simulink model "AxialPump_23a"  (R2023a)
settings: Solver=FixedStepAuto  StartTime=0.0  StopTime=t_cycle  FixedStep=1e-8  RelTol=1e-3  EnableMultiTasking=on
InitFcn:
  | %% Outlet
  | % Parameters
  | d_cyl = 8e-3;                                   % Diameter of each piston
  | r_p = 20e-3;                                    % Piston pitch radius
  | A_cyl = 0.25 * pi * d_cyl^2;                    % Area of each piston
  | omega_rpm = 3600;                               % Rotational speed of pump
  | omega = (2*pi/60) * omega_rpm;                  % Angular speed of pump
  | beta = 1.6e9;                                   % Bulk Modulus
  | P1 = 21e6;                                      % Outlet pressure
  | S = 15e-3;                                      % Stroke length
  | Cd = 0.6;                                       % Coefficient of discharge
  | rho = 870;                                      % Density
  | P_T = 101325;                                   % Tank pressure
  | P_P = 21e6;                                     % System pressure
  | c = 80e-6;                                      % Piston-barrel clearance
  | meu = 0.1;                                      % Steel-steel (lubricated) coefficient of friction
  | r2_r1 = 1.6;                                    % Slipper radii ratio
  | r1 = d_cyl/2;
  | do = 0.1e-3;                                    % Slipper orifice opening
  | 
  | % Time parameters
  | theta_cycle = 2 * pi;
  | t_cycle = theta_cycle / omega;
  | theta_t = 2 * asin(d_cyl/(4*r_p));
  | t_t = theta_t/omega;
  | theta_d = theta_cycle/2 - 2 * theta_t;
  | t_d = theta_d/omega;
  | 
  | t_A_p = [0, 0.5*t_t, t_t, t_t+t_d, 1.5*t_t+t_d, t_cycle];
  | A_p = [0, 0, A_cyl, A_cyl, 0, 0];
  | 
  | t_A_t = [0, 2.5*t_t+t_d, 3*t_t+t_d, 3*t_t+2*t_d, 3.5*t_t+2*t_d, t_cycle];
  | A_t = [0, 0, A_cyl, A_cyl, 0, 0];
  | 
  | % Calculated parameters
  | Vdisp = 0.25 * pi * d_cyl^2 * S;
  | Vo = Vdisp;
libraries: SignalEditorBlockLib x18
(part 2 of 2)

== system AxialPump_23a/Piston 2/Full Throttling Loss (Tank Side) ==
  Pc : Inport
  P_T : Inport  Port=2
  Q_T : Inport  Port=3
  Display : Display
  Integrator : Integrator
  MATLAB Function : MATLAB Function  TreatAsAtomicUnit=on
  Scope : Scope
  " E_ftlts" : Outport
  wires:
  MATLAB Function/1(P_ftlts) -> Scope/1, Integrator/1
  Integrator/1 -> Display/1, " E_ftlts"/1  "E_ftlts"
  Pc/1 -> MATLAB Function/2(Pc)
  P_T/1 -> MATLAB Function/1(P_T)
  Q_T/1 -> MATLAB Function/3(Q_T)

== system AxialPump_23a/Piston 2/Hydrostatic Bearing Loss ==
  Pc : Inport
  Constant : Constant  Value=Cd
  Constant1 : Constant  Value=r2_r1
  Constant2 : Constant  Value=r1
  Constant3 : Constant  Value=do
  Constant4 : Constant  Value=d_cyl
  Constant5 : Constant  Value=rho
  Display : Display
  Integrator : Integrator
  MATLAB Function : MATLAB Function  TreatAsAtomicUnit=on
  Product : Product
  Ehbl : Outport
  wires:
  Constant1/1 -> MATLAB Function/2(r2_r1)
  Constant/1 -> MATLAB Function/6(Cd)
  Constant4/1 -> MATLAB Function/5(d_cyl)
  Constant3/1 -> MATLAB Function/4(do)
  Constant2/1 -> MATLAB Function/3(r1)
  Pc/1 -> Product/2, MATLAB Function/7(Pc)
  MATLAB Function/1(Qhbl) -> Product/1
  Product/1 -> Integrator/1  "Phbl"
  Integrator/1 -> Display/1, Ehbl/1
  Constant5/1 -> MATLAB Function/1(rho)

== system AxialPump_23a/Piston 2/Qleak ==
  Pc : Inport
  Constant : Constant  Value=P_T
  Constant1 : Constant  Value=d_cyl
  Constant2 : Constant  Value=c
  Constant3 : Constant  Value=meu
  Constant4 : Constant  Value=S
  Display : Display
  Integrator2 : Integrator
  MATLAB Function : MATLAB Function  TreatAsAtomicUnit=on
  Product1 : Product
  Eleak : Outport
  wires:
  Constant/1 -> MATLAB Function/2(P_T)
  Constant1/1 -> MATLAB Function/3(d_cyl)
  Constant2/1 -> MATLAB Function/4(c)
  Constant3/1 -> MATLAB Function/5(meu)
  Constant4/1 -> MATLAB Function/6(S)
  Pc/1 -> MATLAB Function/1(Pc), Product1/2
  MATLAB Function/1(Qleak) -> Product1/1
  Integrator2/1 -> Display/1, Eleak/1
  Product1/1 -> Integrator2/1  "Pleakage"

== system AxialPump_23a/Piston 3/Frictional Energy Loss ==
  Vc_dot : Inport
  Vc : Inport  Port=2
  Constant : Constant  Value=Vo
  Constant1 : Constant  Value=A_cyl
  Constant2 : Constant  Value=S
  Constant3 : Constant  Value=c
  Constant4 : Constant  Value=meu
  Constant5 : Constant  Value=d_cyl
  Frictional Energy Loss : Display
  Gain : Gain  Gain=1/A_cyl
  Integrator : Integrator
  MATLAB Function : MATLAB Function  TreatAsAtomicUnit=on
  Scope : Scope
  Efric : Outport
  wires:
  Integrator/1 -> Frictional Energy Loss/1, Efric/1
  Vc_dot/1 -> Gain/1
  Gain/1 -> MATLAB Function/1(xdot)  "xdot"
  MATLAB Function/1(Pfric) -> Integrator/1  "Pfric"
  MATLAB Function/2(x) -> Scope/1  "x"
  Vc/1 -> MATLAB Function/2(Vc)
  Constant/1 -> MATLAB Function/3(Vo)
  Constant1/1 -> MATLAB Function/4(A_cyl)
  Constant2/1 -> MATLAB Function/5(S)
  Constant3/1 -> MATLAB Function/6(c)
  Constant4/1 -> MATLAB Function/7(meu)
  Constant5/1 -> MATLAB Function/8(d_cyl)

== system AxialPump_23a/Piston 3/Full Throttling Loss (Pressure Side) ==
  Pc : Inport
  P_P : Inport  Port=2
  Q_P : Inport  Port=3
  Display : Display
  Integrator : Integrator
  MATLAB Function : MATLAB Function  TreatAsAtomicUnit=on
  Scope : Scope
  " E_ftlps" : Outport
  wires:
  MATLAB Function/1(P_ftlps) -> Scope/1, Integrator/1
  Integrator/1 -> Display/1, " E_ftlps"/1  "E_ftlps"
  Pc/1 -> MATLAB Function/1(Pc)
  P_P/1 -> MATLAB Function/2(P_P)
  Q_P/1 -> MATLAB Function/3(Q_P)

== system AxialPump_23a/Piston 3/Full Throttling Loss (Tank Side) ==
  Pc : Inport
  P_T : Inport  Port=2
  Q_T : Inport  Port=3
  Display : Display
  Integrator : Integrator
  MATLAB Function : MATLAB Function  TreatAsAtomicUnit=on
  Scope : Scope
  " E_ftlts" : Outport
  wires:
  MATLAB Function/1(P_ftlts) -> Scope/1, Integrator/1
  Integrator/1 -> Display/1, " E_ftlts"/1  "E_ftlts"
  Pc/1 -> MATLAB Function/2(Pc)
  P_T/1 -> MATLAB Function/1(P_T)
  Q_T/1 -> MATLAB Function/3(Q_T)

== system AxialPump_23a/Piston 3/Hydrostatic Bearing Loss ==
  Pc : Inport
  Constant : Constant  Value=Cd
  Constant1 : Constant  Value=r2_r1
  Constant2 : Constant  Value=r1
  Constant3 : Constant  Value=do
  Constant4 : Constant  Value=d_cyl
  Constant5 : Constant  Value=rho
  Display : Display
  Integrator : Integrator
  MATLAB Function : MATLAB Function  TreatAsAtomicUnit=on
  Product : Product
  Ehbl : Outport
  wires:
  Constant1/1 -> MATLAB Function/2(r2_r1)
  Constant/1 -> MATLAB Function/6(Cd)
  Constant4/1 -> MATLAB Function/5(d_cyl)
  Constant3/1 -> MATLAB Function/4(do)
  Constant2/1 -> MATLAB Function/3(r1)
  Pc/1 -> Product/2, MATLAB Function/7(Pc)
  MATLAB Function/1(Qhbl) -> Product/1
  Product/1 -> Integrator/1  "Phbl"
  Integrator/1 -> Display/1, Ehbl/1
  Constant5/1 -> MATLAB Function/1(rho)

== system AxialPump_23a/Piston 3/Qleak ==
  Pc : Inport
  Constant : Constant  Value=P_T
  Constant1 : Constant  Value=d_cyl
  Constant2 : Constant  Value=c
  Constant3 : Constant  Value=meu
  Constant4 : Constant  Value=S
  Display : Display
  Integrator2 : Integrator
  MATLAB Function : MATLAB Function  TreatAsAtomicUnit=on
  Product1 : Product
  Eleak : Outport
  wires:
  Constant/1 -> MATLAB Function/2(P_T)
  Constant1/1 -> MATLAB Function/3(d_cyl)
  Constant2/1 -> MATLAB Function/4(c)
  Constant3/1 -> MATLAB Function/5(meu)
  Constant4/1 -> MATLAB Function/6(S)
  Pc/1 -> MATLAB Function/1(Pc), Product1/2
  MATLAB Function/1(Qleak) -> Product1/1
  Integrator2/1 -> Display/1, Eleak/1
  Product1/1 -> Integrator2/1  "Pleakage"

== system AxialPump_23a/Piston 4/Frictional Energy Loss ==
  Vc_dot : Inport
  Vc : Inport  Port=2
  Constant : Constant  Value=Vo
  Constant1 : Constant  Value=A_cyl
  Constant2 : Constant  Value=S
  Constant3 : Constant  Value=c
  Constant4 : Constant  Value=meu
  Constant5 : Constant  Value=d_cyl
  Frictional Energy Loss : Display
  Gain : Gain  Gain=1/A_cyl
  Integrator : Integrator
  MATLAB Function : MATLAB Function  TreatAsAtomicUnit=on
  Scope : Scope
  Efric : Outport
  wires:
  Integrator/1 -> Frictional Energy Loss/1, Efric/1
  Vc_dot/1 -> Gain/1
  Gain/1 -> MATLAB Function/1(xdot)  "xdot"
  MATLAB Function/1(Pfric) -> Integrator/1  "Pfric"
  MATLAB Function/2(x) -> Scope/1  "x"
  Vc/1 -> MATLAB Function/2(Vc)
  Constant/1 -> MATLAB Function/3(Vo)
  Constant1/1 -> MATLAB Function/4(A_cyl)
  Constant2/1 -> MATLAB Function/5(S)
  Constant3/1 -> MATLAB Function/6(c)
  Constant4/1 -> MATLAB Function/7(meu)
  Constant5/1 -> MATLAB Function/8(d_cyl)

== system AxialPump_23a/Piston 4/Full Throttling Loss (Pressure Side) ==
  Pc : Inport
  P_P : Inport  Port=2
  Q_P : Inport  Port=3
  Display : Display
  Integrator : Integrator
  MATLAB Function : MATLAB Function  TreatAsAtomicUnit=on
  Scope : Scope
  " E_ftlps" : Outport
  wires:
  MATLAB Function/1(P_ftlps) -> Scope/1, Integrator/1
  Integrator/1 -> Display/1, " E_ftlps"/1  "E_ftlps"
  Pc/1 -> MATLAB Function/1(Pc)
  P_P/1 -> MATLAB Function/2(P_P)
  Q_P/1 -> MATLAB Function/3(Q_P)

== system AxialPump_23a/Piston 4/Full Throttling Loss (Tank Side) ==
  Pc : Inport
  P_T : Inport  Port=2
  Q_T : Inport  Port=3
  Display : Display
  Integrator : Integrator
  MATLAB Function : MATLAB Function  TreatAsAtomicUnit=on
  Scope : Scope
  " E_ftlts" : Outport
  wires:
  MATLAB Function/1(P_ftlts) -> Scope/1, Integrator/1
  Integrator/1 -> Display/1, " E_ftlts"/1  "E_ftlts"
  Pc/1 -> MATLAB Function/2(Pc)
  P_T/1 -> MATLAB Function/1(P_T)
  Q_T/1 -> MATLAB Function/3(Q_T)

== system AxialPump_23a/Piston 4/Hydrostatic Bearing Loss ==
  Pc : Inport
  Constant : Constant  Value=Cd
  Constant1 : Constant  Value=r2_r1
  Constant2 : Constant  Value=r1
  Constant3 : Constant  Value=do
  Constant4 : Constant  Value=d_cyl
  Constant5 : Constant  Value=rho
  Display : Display
  Integrator : Integrator
  MATLAB Function : MATLAB Function  TreatAsAtomicUnit=on
  Product : Product
  Ehbl : Outport
  wires:
  Constant1/1 -> MATLAB Function/2(r2_r1)
  Constant/1 -> MATLAB Function/6(Cd)
  Constant4/1 -> MATLAB Function/5(d_cyl)
  Constant3/1 -> MATLAB Function/4(do)
  Constant2/1 -> MATLAB Function/3(r1)
  Pc/1 -> Product/2, MATLAB Function/7(Pc)
  MATLAB Function/1(Qhbl) -> Product/1
  Product/1 -> Integrator/1  "Phbl"
  Integrator/1 -> Display/1, Ehbl/1
  Constant5/1 -> MATLAB Function/1(rho)

== system AxialPump_23a/Piston 4/Qleak ==
  Pc : Inport
  Constant : Constant  Value=P_T
  Constant1 : Constant  Value=d_cyl
  Constant2 : Constant  Value=c
  Constant3 : Constant  Value=meu
  Constant4 : Constant  Value=S
  Display : Display
  Integrator2 : Integrator
  MATLAB Function : MATLAB Function  TreatAsAtomicUnit=on
  Product1 : Product
  Eleak : Outport
  wires:
  Constant/1 -> MATLAB Function/2(P_T)
  Constant1/1 -> MATLAB Function/3(d_cyl)
  Constant2/1 -> MATLAB Function/4(c)
  Constant3/1 -> MATLAB Function/5(meu)
  Constant4/1 -> MATLAB Function/6(S)
  Pc/1 -> MATLAB Function/1(Pc), Product1/2
  MATLAB Function/1(Qleak) -> Product1/1
  Integrator2/1 -> Display/1, Eleak/1
  Product1/1 -> Integrator2/1  "Pleakage"

== system AxialPump_23a/Piston 5/Frictional Energy Loss ==
  Vc_dot : Inport
  Vc : Inport  Port=2
  Constant : Constant  Value=Vo
  Constant1 : Constant  Value=A_cyl
  Constant2 : Constant  Value=S
  Constant3 : Constant  Value=c
  Constant4 : Constant  Value=meu
  Constant5 : Constant  Value=d_cyl
  Frictional Energy Loss : Display
  Gain : Gain  Gain=1/A_cyl
  Integrator : Integrator
  MATLAB Function : MATLAB Function  TreatAsAtomicUnit=on
  Scope : Scope
  Efric : Outport
  wires:
  Integrator/1 -> Frictional Energy Loss/1, Efric/1
  Vc_dot/1 -> Gain/1
  Gain/1 -> MATLAB Function/1(xdot)  "xdot"
  MATLAB Function/1(Pfric) -> Integrator/1  "Pfric"
  MATLAB Function/2(x) -> Scope/1  "x"
  Vc/1 -> MATLAB Function/2(Vc)
  Constant/1 -> MATLAB Function/3(Vo)
  Constant1/1 -> MATLAB Function/4(A_cyl)
  Constant2/1 -> MATLAB Function/5(S)
  Constant3/1 -> MATLAB Function/6(c)
  Constant4/1 -> MATLAB Function/7(meu)
  Constant5/1 -> MATLAB Function/8(d_cyl)

== system AxialPump_23a/Piston 5/Full Throttling Loss (Pressure Side) ==
  Pc : Inport
  P_P : Inport  Port=2
  Q_P : Inport  Port=3
  Display : Display
  Integrator : Integrator
  MATLAB Function : MATLAB Function  TreatAsAtomicUnit=on
  Scope : Scope
  " E_ftlps" : Outport
  wires:
  MATLAB Function/1(P_ftlps) -> Scope/1, Integrator/1
  Integrator/1 -> Display/1, " E_ftlps"/1  "E_ftlps"
  Pc/1 -> MATLAB Function/1(Pc)
  P_P/1 -> MATLAB Function/2(P_P)
  Q_P/1 -> MATLAB Function/3(Q_P)

== system AxialPump_23a/Piston 5/Full Throttling Loss (Tank Side) ==
  Pc : Inport
  P_T : Inport  Port=2
  Q_T : Inport  Port=3
  Display : Display
  Integrator : Integrator
  MATLAB Function : MATLAB Function  TreatAsAtomicUnit=on
  Scope : Scope
  " E_ftlts" : Outport
  wires:
  MATLAB Function/1(P_ftlts) -> Scope/1, Integrator/1
  Integrator/1 -> Display/1, " E_ftlts"/1  "E_ftlts"
  Pc/1 -> MATLAB Function/2(Pc)
  P_T/1 -> MATLAB Function/1(P_T)
  Q_T/1 -> MATLAB Function/3(Q_T)

== system AxialPump_23a/Piston 5/Hydrostatic Bearing Loss ==
  Pc : Inport
  Constant : Constant  Value=Cd
  Constant1 : Constant  Value=r2_r1
  Constant2 : Constant  Value=r1
  Constant3 : Constant  Value=do
  Constant4 : Constant  Value=d_cyl
  Constant5 : Constant  Value=rho
  Display : Display
  Integrator : Integrator
  MATLAB Function : MATLAB Function  TreatAsAtomicUnit=on
  Product : Product
  Ehbl : Outport
  wires:
  Constant1/1 -> MATLAB Function/2(r2_r1)
  Constant/1 -> MATLAB Function/6(Cd)
  Constant4/1 -> MATLAB Function/5(d_cyl)
  Constant3/1 -> MATLAB Function/4(do)
  Constant2/1 -> MATLAB Function/3(r1)
  Pc/1 -> Product/2, MATLAB Function/7(Pc)
  MATLAB Function/1(Qhbl) -> Product/1
  Product/1 -> Integrator/1  "Phbl"
  Integrator/1 -> Display/1, Ehbl/1
  Constant5/1 -> MATLAB Function/1(rho)

== system AxialPump_23a/Piston 5/Qleak ==
  Pc : Inport
  Constant : Constant  Value=P_T
  Constant1 : Constant  Value=d_cyl
  Constant2 : Constant  Value=c
  Constant3 : Constant  Value=meu
  Constant4 : Constant  Value=S
  Display : Display
  Integrator2 : Integrator
  MATLAB Function : MATLAB Function  TreatAsAtomicUnit=on
  Product1 : Product
  Eleak : Outport
  wires:
  Constant/1 -> MATLAB Function/2(P_T)
  Constant1/1 -> MATLAB Function/3(d_cyl)
  Constant2/1 -> MATLAB Function/4(c)
  Constant3/1 -> MATLAB Function/5(meu)
  Constant4/1 -> MATLAB Function/6(S)
  Pc/1 -> MATLAB Function/1(Pc), Product1/2
  MATLAB Function/1(Qleak) -> Product1/1
  Integrator2/1 -> Display/1, Eleak/1
  Product1/1 -> Integrator2/1  "Pleakage"

== system AxialPump_23a/Piston 6/Frictional Energy Loss ==
  Vc_dot : Inport
  Vc : Inport  Port=2
  Constant : Constant  Value=Vo
  Constant1 : Constant  Value=A_cyl
  Constant2 : Constant  Value=S
  Constant3 : Constant  Value=c
  Constant4 : Constant  Value=meu
  Constant5 : Constant  Value=d_cyl
  Frictional Energy Loss : Display
  Gain : Gain  Gain=1/A_cyl
  Integrator : Integrator
  MATLAB Function : MATLAB Function  TreatAsAtomicUnit=on
  Scope : Scope
  Efric : Outport
  wires:
  Integrator/1 -> Frictional Energy Loss/1, Efric/1
  Vc_dot/1 -> Gain/1
  Gain/1 -> MATLAB Function/1(xdot)  "xdot"
  MATLAB Function/1(Pfric) -> Integrator/1  "Pfric"
  MATLAB Function/2(x) -> Scope/1  "x"
  Vc/1 -> MATLAB Function/2(Vc)
  Constant/1 -> MATLAB Function/3(Vo)
  Constant1/1 -> MATLAB Function/4(A_cyl)
  Constant2/1 -> MATLAB Function/5(S)
  Constant3/1 -> MATLAB Function/6(c)
  Constant4/1 -> MATLAB Function/7(meu)
  Constant5/1 -> MATLAB Function/8(d_cyl)

== system AxialPump_23a/Piston 6/Full Throttling Loss (Pressure Side) ==
  Pc : Inport
  P_P : Inport  Port=2
  Q_P : Inport  Port=3
  Display : Display
  Integrator : Integrator
  MATLAB Function : MATLAB Function  TreatAsAtomicUnit=on
  Scope : Scope
  " E_ftlps" : Outport
  wires:
  MATLAB Function/1(P_ftlps) -> Scope/1, Integrator/1
  Integrator/1 -> Display/1, " E_ftlps"/1  "E_ftlps"
  Pc/1 -> MATLAB Function/1(Pc)
  P_P/1 -> MATLAB Function/2(P_P)
  Q_P/1 -> MATLAB Function/3(Q_P)

== system AxialPump_23a/Piston 6/Full Throttling Loss (Tank Side) ==
  Pc : Inport
  P_T : Inport  Port=2
  Q_T : Inport  Port=3
  Display : Display
  Integrator : Integrator
  MATLAB Function : MATLAB Function  TreatAsAtomicUnit=on
  Scope : Scope
  " E_ftlts" : Outport
  wires:
  MATLAB Function/1(P_ftlts) -> Scope/1, Integrator/1
  Integrator/1 -> Display/1, " E_ftlts"/1  "E_ftlts"
  Pc/1 -> MATLAB Function/2(Pc)
  P_T/1 -> MATLAB Function/1(P_T)
  Q_T/1 -> MATLAB Function/3(Q_T)

== system AxialPump_23a/Piston 6/Hydrostatic Bearing Loss ==
  Pc : Inport
  Constant : Constant  Value=Cd
  Constant1 : Constant  Value=r2_r1
  Constant2 : Constant  Value=r1
  Constant3 : Constant  Value=do
  Constant4 : Constant  Value=d_cyl
  Constant5 : Constant  Value=rho
  Display : Display
  Integrator : Integrator
  MATLAB Function : MATLAB Function  TreatAsAtomicUnit=on
  Product : Product
  Ehbl : Outport
  wires:
  Constant1/1 -> MATLAB Function/2(r2_r1)
  Constant/1 -> MATLAB Function/6(Cd)
  Constant4/1 -> MATLAB Function/5(d_cyl)
  Constant3/1 -> MATLAB Function/4(do)
  Constant2/1 -> MATLAB Function/3(r1)
  Pc/1 -> Product/2, MATLAB Function/7(Pc)
  MATLAB Function/1(Qhbl) -> Product/1
  Product/1 -> Integrator/1  "Phbl"
  Integrator/1 -> Display/1, Ehbl/1
  Constant5/1 -> MATLAB Function/1(rho)

== system AxialPump_23a/Piston 6/Qleak ==
  Pc : Inport
  Constant : Constant  Value=P_T
  Constant1 : Constant  Value=d_cyl
  Constant2 : Constant  Value=c
  Constant3 : Constant  Value=meu
  Constant4 : Constant  Value=S
  Display : Display
  Integrator2 : Integrator
  MATLAB Function : MATLAB Function  TreatAsAtomicUnit=on
  Product1 : Product
  Eleak : Outport
  wires:
  Constant/1 -> MATLAB Function/2(P_T)
  Constant1/1 -> MATLAB Function/3(d_cyl)
  Constant2/1 -> MATLAB Function/4(c)
  Constant3/1 -> MATLAB Function/5(meu)
  Constant4/1 -> MATLAB Function/6(S)
  Pc/1 -> MATLAB Function/1(Pc), Product1/2
  MATLAB Function/1(Qleak) -> Product1/1
  Integrator2/1 -> Display/1, Eleak/1
  Product1/1 -> Integrator2/1  "Pleakage"

== system AxialPump_23a/Piston 7/Frictional Energy Loss ==
  Vc_dot : Inport
  Vc : Inport  Port=2
  Constant : Constant  Value=Vo
  Constant1 : Constant  Value=A_cyl
  Constant2 : Constant  Value=S
  Constant3 : Constant  Value=c
  Constant4 : Constant  Value=meu
  Constant5 : Constant  Value=d_cyl
  Frictional Energy Loss : Display
  Gain : Gain  Gain=1/A_cyl
  Integrator : Integrator
  MATLAB Function : MATLAB Function  TreatAsAtomicUnit=on
  Scope : Scope
  Efric : Outport
  wires:
  Integrator/1 -> Frictional Energy Loss/1, Efric/1
  Vc_dot/1 -> Gain/1
  Gain/1 -> MATLAB Function/1(xdot)  "xdot"
  MATLAB Function/1(Pfric) -> Integrator/1  "Pfric"
  MATLAB Function/2(x) -> Scope/1  "x"
  Vc/1 -> MATLAB Function/2(Vc)
  Constant/1 -> MATLAB Function/3(Vo)
  Constant1/1 -> MATLAB Function/4(A_cyl)
  Constant2/1 -> MATLAB Function/5(S)
  Constant3/1 -> MATLAB Function/6(c)
  Constant4/1 -> MATLAB Function/7(meu)
  Constant5/1 -> MATLAB Function/8(d_cyl)

== system AxialPump_23a/Piston 7/Full Throttling Loss (Pressure Side) ==
  Pc : Inport
  P_P : Inport  Port=2
  Q_P : Inport  Port=3
  Display : Display
  Integrator : Integrator
  MATLAB Function : MATLAB Function  TreatAsAtomicUnit=on
  Scope : Scope
  " E_ftlps" : Outport
  wires:
  MATLAB Function/1(P_ftlps) -> Scope/1, Integrator/1
  Integrator/1 -> Display/1, " E_ftlps"/1  "E_ftlps"
  Pc/1 -> MATLAB Function/1(Pc)
  P_P/1 -> MATLAB Function/2(P_P)
  Q_P/1 -> MATLAB Function/3(Q_P)

== system AxialPump_23a/Piston 7/Full Throttling Loss (Tank Side) ==
  Pc : Inport
  P_T : Inport  Port=2
  Q_T : Inport  Port=3
  Display : Display
  Integrator : Integrator
  MATLAB Function : MATLAB Function  TreatAsAtomicUnit=on
  Scope : Scope
  " E_ftlts" : Outport
  wires:
  MATLAB Function/1(P_ftlts) -> Scope/1, Integrator/1
  Integrator/1 -> Display/1, " E_ftlts"/1  "E_ftlts"
  Pc/1 -> MATLAB Function/2(Pc)
  P_T/1 -> MATLAB Function/1(P_T)
  Q_T/1 -> MATLAB Function/3(Q_T)

== system AxialPump_23a/Piston 7/Hydrostatic Bearing Loss ==
  Pc : Inport
  Constant : Constant  Value=Cd
  Constant1 : Constant  Value=r2_r1
  Constant2 : Constant  Value=r1
  Constant3 : Constant  Value=do
  Constant4 : Constant  Value=d_cyl
  Constant5 : Constant  Value=rho
  Display : Display
  Integrator : Integrator
  MATLAB Function : MATLAB Function  TreatAsAtomicUnit=on
  Product : Product
  Ehbl : Outport
  wires:
  Constant1/1 -> MATLAB Function/2(r2_r1)
  Constant/1 -> MATLAB Function/6(Cd)
  Constant4/1 -> MATLAB Function/5(d_cyl)
  Constant3/1 -> MATLAB Function/4(do)
  Constant2/1 -> MATLAB Function/3(r1)
  Pc/1 -> Product/2, MATLAB Function/7(Pc)
  MATLAB Function/1(Qhbl) -> Product/1
  Product/1 -> Integrator/1  "Phbl"
  Integrator/1 -> Display/1, Ehbl/1
  Constant5/1 -> MATLAB Function/1(rho)

== system AxialPump_23a/Piston 7/Qleak ==
  Pc : Inport
  Constant : Constant  Value=P_T
  Constant1 : Constant  Value=d_cyl
  Constant2 : Constant  Value=c
  Constant3 : Constant  Value=meu
  Constant4 : Constant  Value=S
  Display : Display
  Integrator2 : Integrator
  MATLAB Function : MATLAB Function  TreatAsAtomicUnit=on
  Product1 : Product
  Eleak : Outport
  wires:
  Constant/1 -> MATLAB Function/2(P_T)
  Constant1/1 -> MATLAB Function/3(d_cyl)
  Constant2/1 -> MATLAB Function/4(c)
  Constant3/1 -> MATLAB Function/5(meu)
  Constant4/1 -> MATLAB Function/6(S)
  Pc/1 -> MATLAB Function/1(Pc), Product1/2
  MATLAB Function/1(Qleak) -> Product1/1
  Integrator2/1 -> Display/1, Eleak/1
  Product1/1 -> Integrator2/1  "Pleakage"

== system AxialPump_23a/Piston 8/Frictional Energy Loss ==
  Vc_dot : Inport
  Vc : Inport  Port=2
  Constant : Constant  Value=Vo
  Constant1 : Constant  Value=A_cyl
  Constant2 : Constant  Value=S
  Constant3 : Constant  Value=c
  Constant4 : Constant  Value=meu
  Constant5 : Constant  Value=d_cyl
  Frictional Energy Loss : Display
  Gain : Gain  Gain=1/A_cyl
  Integrator : Integrator
  MATLAB Function : MATLAB Function  TreatAsAtomicUnit=on
  Scope : Scope
  Efric : Outport
  wires:
  Integrator/1 -> Frictional Energy Loss/1, Efric/1
  Vc_dot/1 -> Gain/1
  Gain/1 -> MATLAB Function/1(xdot)  "xdot"
  MATLAB Function/1(Pfric) -> Integrator/1  "Pfric"
  MATLAB Function/2(x) -> Scope/1  "x"
  Vc/1 -> MATLAB Function/2(Vc)
  Constant/1 -> MATLAB Function/3(Vo)
  Constant1/1 -> MATLAB Function/4(A_cyl)
  Constant2/1 -> MATLAB Function/5(S)
  Constant3/1 -> MATLAB Function/6(c)
  Constant4/1 -> MATLAB Function/7(meu)
  Constant5/1 -> MATLAB Function/8(d_cyl)

== system AxialPump_23a/Piston 8/Full Throttling Loss (Pressure Side) ==
  Pc : Inport
  P_P : Inport  Port=2
  Q_P : Inport  Port=3
  Display : Display
  Integrator : Integrator
  MATLAB Function : MATLAB Function  TreatAsAtomicUnit=on
  Scope : Scope
  " E_ftlps" : Outport
  wires:
  MATLAB Function/1(P_ftlps) -> Scope/1, Integrator/1
  Integrator/1 -> Display/1, " E_ftlps"/1  "E_ftlps"
  Pc/1 -> MATLAB Function/1(Pc)
  P_P/1 -> MATLAB Function/2(P_P)
  Q_P/1 -> MATLAB Function/3(Q_P)

== system AxialPump_23a/Piston 8/Full Throttling Loss (Tank Side) ==
  Pc : Inport
  P_T : Inport  Port=2
  Q_T : Inport  Port=3
  Display : Display
  Integrator : Integrator
  MATLAB Function : MATLAB Function  TreatAsAtomicUnit=on
  Scope : Scope
  " E_ftlts" : Outport
  wires:
  MATLAB Function/1(P_ftlts) -> Scope/1, Integrator/1
  Integrator/1 -> Display/1, " E_ftlts"/1  "E_ftlts"
  Pc/1 -> MATLAB Function/2(Pc)
  P_T/1 -> MATLAB Function/1(P_T)
  Q_T/1 -> MATLAB Function/3(Q_T)

== system AxialPump_23a/Piston 8/Hydrostatic Bearing Loss ==
  Pc : Inport
  Constant : Constant  Value=Cd
  Constant1 : Constant  Value=r2_r1
  Constant2 : Constant  Value=r1
  Constant3 : Constant  Value=do
  Constant4 : Constant  Value=d_cyl
  Constant5 : Constant  Value=rho
  Display : Display
  Integrator : Integrator
  MATLAB Function : MATLAB Function  TreatAsAtomicUnit=on
  Product : Product
  Ehbl : Outport
  wires:
  Constant1/1 -> MATLAB Function/2(r2_r1)
  Constant/1 -> MATLAB Function/6(Cd)
  Constant4/1 -> MATLAB Function/5(d_cyl)
  Constant3/1 -> MATLAB Function/4(do)
  Constant2/1 -> MATLAB Function/3(r1)
  Pc/1 -> Product/2, MATLAB Function/7(Pc)
  MATLAB Function/1(Qhbl) -> Product/1
  Product/1 -> Integrator/1  "Phbl"
  Integrator/1 -> Display/1, Ehbl/1
  Constant5/1 -> MATLAB Function/1(rho)

== system AxialPump_23a/Piston 8/Qleak ==
  Pc : Inport
  Constant : Constant  Value=P_T
  Constant1 : Constant  Value=d_cyl
  Constant2 : Constant  Value=c
  Constant3 : Constant  Value=meu
  Constant4 : Constant  Value=S
  Display : Display
  Integrator2 : Integrator
  MATLAB Function : MATLAB Function  TreatAsAtomicUnit=on
  Product1 : Product
  Eleak : Outport
  wires:
  Constant/1 -> MATLAB Function/2(P_T)
  Constant1/1 -> MATLAB Function/3(d_cyl)
  Constant2/1 -> MATLAB Function/4(c)
  Constant3/1 -> MATLAB Function/5(meu)
  Constant4/1 -> MATLAB Function/6(S)
  Pc/1 -> MATLAB Function/1(Pc), Product1/2
  MATLAB Function/1(Qleak) -> Product1/1
  Integrator2/1 -> Display/1, Eleak/1
  Product1/1 -> Integrator2/1  "Pleakage"

== system AxialPump_23a/Piston 9/Frictional Energy Loss ==
  Vc_dot : Inport
  Vc : Inport  Port=2
  Constant : Constant  Value=Vo
  Constant1 : Constant  Value=A_cyl
  Constant2 : Constant  Value=S
  Constant3 : Constant  Value=c
  Constant4 : Constant  Value=meu
  Constant5 : Constant  Value=d_cyl
  Frictional Energy Loss : Display
  Gain : Gain  Gain=1/A_cyl
  Integrator : Integrator
  MATLAB Function : MATLAB Function  TreatAsAtomicUnit=on
  Scope : Scope
  Efric : Outport
  wires:
  Integrator/1 -> Frictional Energy Loss/1, Efric/1
  Vc_dot/1 -> Gain/1
  Gain/1 -> MATLAB Function/1(xdot)  "xdot"
  MATLAB Function/1(Pfric) -> Integrator/1  "Pfric"
  MATLAB Function/2(x) -> Scope/1  "x"
  Vc/1 -> MATLAB Function/2(Vc)
  Constant/1 -> MATLAB Function/3(Vo)
  Constant1/1 -> MATLAB Function/4(A_cyl)
  Constant2/1 -> MATLAB Function/5(S)
  Constant3/1 -> MATLAB Function/6(c)
  Constant4/1 -> MATLAB Function/7(meu)
  Constant5/1 -> MATLAB Function/8(d_cyl)

== system AxialPump_23a/Piston 9/Full Throttling Loss (Pressure Side) ==
  Pc : Inport
  P_P : Inport  Port=2
  Q_P : Inport  Port=3
  Display : Display
  Integrator : Integrator
  MATLAB Function : MATLAB Function  TreatAsAtomicUnit=on
  Scope : Scope
  " E_ftlps" : Outport
  wires:
  MATLAB Function/1(P_ftlps) -> Scope/1, Integrator/1
  Integrator/1 -> Display/1, " E_ftlps"/1  "E_ftlps"
  Pc/1 -> MATLAB Function/1(Pc)
  P_P/1 -> MATLAB Function/2(P_P)
  Q_P/1 -> MATLAB Function/3(Q_P)

== system AxialPump_23a/Piston 9/Full Throttling Loss (Tank Side) ==
  Pc : Inport
  P_T : Inport  Port=2
  Q_T : Inport  Port=3
  Display : Display
  Integrator : Integrator
  MATLAB Function : MATLAB Function  TreatAsAtomicUnit=on
  Scope : Scope
  " E_ftlts" : Outport
  wires:
  MATLAB Function/1(P_ftlts) -> Scope/1, Integrator/1
  Integrator/1 -> Display/1, " E_ftlts"/1  "E_ftlts"
  Pc/1 -> MATLAB Function/2(Pc)
  P_T/1 -> MATLAB Function/1(P_T)
  Q_T/1 -> MATLAB Function/3(Q_T)

== system AxialPump_23a/Piston 9/Hydrostatic Bearing Loss ==
  Pc : Inport
  Constant : Constant  Value=Cd
  Constant1 : Constant  Value=r2_r1
  Constant2 : Constant  Value=r1
  Constant3 : Constant  Value=do
  Constant4 : Constant  Value=d_cyl
  Constant5 : Constant  Value=rho
  Display : Display
  Integrator : Integrator
  MATLAB Function : MATLAB Function  TreatAsAtomicUnit=on
  Product : Product
  Ehbl : Outport
  wires:
  Constant1/1 -> MATLAB Function/2(r2_r1)
  Constant/1 -> MATLAB Function/6(Cd)
  Constant4/1 -> MATLAB Function/5(d_cyl)
  Constant3/1 -> MATLAB Function/4(do)
  Constant2/1 -> MATLAB Function/3(r1)
  Pc/1 -> Product/2, MATLAB Function/7(Pc)
  MATLAB Function/1(Qhbl) -> Product/1
  Product/1 -> Integrator/1  "Phbl"
  Integrator/1 -> Display/1, Ehbl/1
  Constant5/1 -> MATLAB Function/1(rho)

== system AxialPump_23a/Piston 9/Qleak ==
  Pc : Inport
  Constant : Constant  Value=P_T
  Constant1 : Constant  Value=d_cyl
  Constant2 : Constant  Value=c
  Constant3 : Constant  Value=meu
  Constant4 : Constant  Value=S
  Display : Display
  Integrator2 : Integrator
  MATLAB Function : MATLAB Function  TreatAsAtomicUnit=on
  Product1 : Product
  Eleak : Outport
  wires:
  Constant/1 -> MATLAB Function/2(P_T)
  Constant1/1 -> MATLAB Function/3(d_cyl)
  Constant2/1 -> MATLAB Function/4(c)
  Constant3/1 -> MATLAB Function/5(meu)
  Constant4/1 -> MATLAB Function/6(S)
  Pc/1 -> MATLAB Function/1(Pc), Product1/2
  MATLAB Function/1(Qleak) -> Product1/1
  Integrator2/1 -> Display/1, Eleak/1
  Product1/1 -> Integrator2/1  "Pleakage"

== matlab function AxialPump_23a/Piston 1/Full Throttling Loss (Tank Side)/MATLAB Function ==
  data: P_T input; Pc input; P_ftlts output; Q_T input
function P_ftlts = fcn(P_T, Pc, Q_T)

P_ftlts = (P_T - Pc) * Q_T;

== matlab function AxialPump_23a/Piston 2/Compressibility Function ==
  data: Vc_dot input; Pc_dot output; Q_T input; Q_P input; beta input; Vc input
function Pc_dot = fcn(Vc_dot, Q_T, Q_P, beta, Vc)

Pc_dot = (beta/Vc) * (Q_T - Q_P - Vc_dot);

== matlab function AxialPump_23a/Piston 2/Frictional Energy Loss/MATLAB Function ==
  data: xdot input; Pfric output; x output; Vc input; Vo input; A_cyl input; S input; c input; meu input; d_cyl input
function [Pfric, x] = fcn(xdot, Vc, Vo, A_cyl, S, c, meu, d_cyl)

x = (Vc - Vo)/A_cyl;
Pfric = (pi*d_cyl*(S-x)*meu*xdot^2)/c;

== matlab function AxialPump_23a/Piston 2/Full Throttling Loss (Pressure Side)/MATLAB Function ==
  data: Pc input; P_ftlps output; P_P input; Q_P input
function P_ftlps = fcn(Pc, P_P, Q_P)

P_ftlps = (Pc - P_P) * Q_P;

== matlab function AxialPump_23a/Piston 2/Full Throttling Loss (Tank Side)/MATLAB Function ==
  data: P_T input; Pc input; P_ftlts output; Q_T input
function P_ftlts = fcn(P_T, Pc, Q_T)

P_ftlts = (P_T - Pc) * Q_T;

== matlab function AxialPump_23a/Piston 2/Hydrostatic Bearing Loss/MATLAB Function ==
  data: rho input; r2_r1 input; Qhbl output; r1 input; do input; d_cyl input; Cd input; Pc input
function Qhbl = fcn(rho, r2_r1, r1, do, d_cyl, Cd, Pc)

F_H = 0.25*Pc*pi*d_cyl^2;
Pp = (2*log(r2_r1)*F_H)/(((r2_r1)^2-1)*pi*r1^2);
Qhbl = 0.25*Cd*do^2*sqrt((2/rho)*abs(Pc-Pp))*sign(Pc-Pp);

== matlab function AxialPump_23a/Piston 2/Pressure Side Flow Rate ==
  data: A_P input; Pc input; P_P input; Cd input; rho input; Q_P output
function Q_P = fcn(A_P, Pc, P_P, Cd, rho)

Q_P = Cd*A_P*sqrt((2/rho)*abs(Pc-P_P))*sign(Pc-P_P);

== matlab function AxialPump_23a/Piston 2/Qleak/MATLAB Function ==
  data: Pc input; Qleak output; P_T input; d_cyl input; c input; meu input; S input
function Qleak = fcn(Pc, P_T, d_cyl, c, meu, S)

Qleak = ((0.25*pi*d_cyl^2)*c^3*(Pc-P_T))/(12*meu*S);

== matlab function AxialPump_23a/Piston 2/Tank Side Flow Rate ==
  data: A_T input; Q_T output; Pc input; P_T input; Cd input; rho input
function Q_T = fcn(A_T, Pc, P_T, Cd, rho)

Q_T = Cd*A_T*sqrt((2/rho)*abs(P_T-Pc))*sign(P_T-Pc);

== matlab function AxialPump_23a/Piston 1/Tank Side Flow Rate ==
  data: A_T input; Q_T output; Pc input; P_T input; Cd input; rho input
function Q_T = fcn(A_T, Pc, P_T, Cd, rho)

Q_T = Cd*A_T*sqrt((2/rho)*abs(P_T-Pc))*sign(P_T-Pc);

== matlab function AxialPump_23a/Piston 3/Compressibility Function ==
  data: Vc_dot input; Pc_dot output; Q_T input; Q_P input; beta input; Vc input
function Pc_dot = fcn(Vc_dot, Q_T, Q_P, beta, Vc)

Pc_dot = (beta/Vc) * (Q_T - Q_P - Vc_dot);

== matlab function AxialPump_23a/Piston 3/Frictional Energy Loss/MATLAB Function ==
  data: xdot input; Pfric output; x output; Vc input; Vo input; A_cyl input; S input; c input; meu input; d_cyl input
function [Pfric, x] = fcn(xdot, Vc, Vo, A_cyl, S, c, meu, d_cyl)

x = (Vc - Vo)/A_cyl;
Pfric = (pi*d_cyl*(S-x)*meu*xdot^2)/c;

== matlab function AxialPump_23a/Piston 3/Full Throttling Loss (Pressure Side)/MATLAB Function ==
  data: Pc input; P_ftlps output; P_P input; Q_P input
function P_ftlps = fcn(Pc, P_P, Q_P)

P_ftlps = (Pc - P_P) * Q_P;

== matlab function AxialPump_23a/Piston 3/Full Throttling Loss (Tank Side)/MATLAB Function ==
  data: P_T input; Pc input; P_ftlts output; Q_T input
function P_ftlts = fcn(P_T, Pc, Q_T)

P_ftlts = (P_T - Pc) * Q_T;

== matlab function AxialPump_23a/Piston 3/Hydrostatic Bearing Loss/MATLAB Function ==
  data: rho input; r2_r1 input; Qhbl output; r1 input; do input; d_cyl input; Cd input; Pc input
function Qhbl = fcn(rho, r2_r1, r1, do, d_cyl, Cd, Pc)

F_H = 0.25*Pc*pi*d_cyl^2;
Pp = (2*log(r2_r1)*F_H)/(((r2_r1)^2-1)*pi*r1^2);
Qhbl = 0.25*Cd*do^2*sqrt((2/rho)*abs(Pc-Pp))*sign(Pc-Pp);

== matlab function AxialPump_23a/Piston 3/Pressure Side Flow Rate ==
  data: A_P input; Pc input; P_P input; Cd input; rho input; Q_P output
function Q_P = fcn(A_P, Pc, P_P, Cd, rho)

Q_P = Cd*A_P*sqrt((2/rho)*abs(Pc-P_P))*sign(Pc-P_P);

== matlab function AxialPump_23a/Piston 3/Qleak/MATLAB Function ==
  data: Pc input; Qleak output; P_T input; d_cyl input; c input; meu input; S input
function Qleak = fcn(Pc, P_T, d_cyl, c, meu, S)

Qleak = ((0.25*pi*d_cyl^2)*c^3*(Pc-P_T))/(12*meu*S);

== matlab function AxialPump_23a/Piston 3/Tank Side Flow Rate ==
  data: A_T input; Q_T output; Pc input; P_T input; Cd input; rho input
function Q_T = fcn(A_T, Pc, P_T, Cd, rho)

Q_T = Cd*A_T*sqrt((2/rho)*abs(P_T-Pc))*sign(P_T-Pc);

== matlab function AxialPump_23a/Piston 4/Compressibility Function ==
  data: Vc_dot input; Pc_dot output; Q_T input; Q_P input; beta input; Vc input
function Pc_dot = fcn(Vc_dot, Q_T, Q_P, beta, Vc)

Pc_dot = (beta/Vc) * (Q_T - Q_P - Vc_dot);

== matlab function AxialPump_23a/Piston 4/Frictional Energy Loss/MATLAB Function ==
  data: xdot input; Pfric output; x output; Vc input; Vo input; A_cyl input; S input; c input; meu input; d_cyl input
function [Pfric, x] = fcn(xdot, Vc, Vo, A_cyl, S, c, meu, d_cyl)

x = (Vc - Vo)/A_cyl;
Pfric = (pi*d_cyl*(S-x)*meu*xdot^2)/c;

== matlab function AxialPump_23a/Piston 1/Compressibility Function ==
  data: Vc_dot input; Pc_dot output; Q_T input; Q_P input; beta input; Vc input
function Pc_dot = fcn(Vc_dot, Q_T, Q_P, beta, Vc)

Pc_dot = (beta/Vc) * (Q_T - Q_P - Vc_dot);

== matlab function AxialPump_23a/Piston 4/Full Throttling Loss (Pressure Side)/MATLAB Function ==
  data: Pc input; P_ftlps output; P_P input; Q_P input
function P_ftlps = fcn(Pc, P_P, Q_P)

P_ftlps = (Pc - P_P) * Q_P;

== matlab function AxialPump_23a/Piston 4/Full Throttling Loss (Tank Side)/MATLAB Function ==
  data: P_T input; Pc input; P_ftlts output; Q_T input
function P_ftlts = fcn(P_T, Pc, Q_T)

P_ftlts = (P_T - Pc) * Q_T;

== matlab function AxialPump_23a/Piston 4/Hydrostatic Bearing Loss/MATLAB Function ==
  data: rho input; r2_r1 input; Qhbl output; r1 input; do input; d_cyl input; Cd input; Pc input
function Qhbl = fcn(rho, r2_r1, r1, do, d_cyl, Cd, Pc)

F_H = 0.25*Pc*pi*d_cyl^2;
Pp = (2*log(r2_r1)*F_H)/(((r2_r1)^2-1)*pi*r1^2);
Qhbl = 0.25*Cd*do^2*sqrt((2/rho)*abs(Pc-Pp))*sign(Pc-Pp);

== matlab function AxialPump_23a/Piston 4/Pressure Side Flow Rate ==
  data: A_P input; Pc input; P_P input; Cd input; rho input; Q_P output
function Q_P = fcn(A_P, Pc, P_P, Cd, rho)

Q_P = Cd*A_P*sqrt((2/rho)*abs(Pc-P_P))*sign(Pc-P_P);

== matlab function AxialPump_23a/Piston 4/Qleak/MATLAB Function ==
  data: Pc input; Qleak output; P_T input; d_cyl input; c input; meu input; S input
function Qleak = fcn(Pc, P_T, d_cyl, c, meu, S)

Qleak = ((0.25*pi*d_cyl^2)*c^3*(Pc-P_T))/(12*meu*S);

== matlab function AxialPump_23a/Piston 4/Tank Side Flow Rate ==
  data: A_T input; Q_T output; Pc input; P_T input; Cd input; rho input
function Q_T = fcn(A_T, Pc, P_T, Cd, rho)

Q_T = Cd*A_T*sqrt((2/rho)*abs(P_T-Pc))*sign(P_T-Pc);

== matlab function AxialPump_23a/Piston 5/Compressibility Function ==
  data: Vc_dot input; Pc_dot output; Q_T input; Q_P input; beta input; Vc input
function Pc_dot = fcn(Vc_dot, Q_T, Q_P, beta, Vc)

Pc_dot = (beta/Vc) * (Q_T - Q_P - Vc_dot);

== matlab function AxialPump_23a/Piston 5/Frictional Energy Loss/MATLAB Function ==
  data: xdot input; Pfric output; x output; Vc input; Vo input; A_cyl input; S input; c input; meu input; d_cyl input
function [Pfric, x] = fcn(xdot, Vc, Vo, A_cyl, S, c, meu, d_cyl)

x = (Vc - Vo)/A_cyl;
Pfric = (pi*d_cyl*(S-x)*meu*xdot^2)/c;

== matlab function AxialPump_23a/Piston 5/Full Throttling Loss (Pressure Side)/MATLAB Function ==
  data: Pc input; P_ftlps output; P_P input; Q_P input
function P_ftlps = fcn(Pc, P_P, Q_P)

P_ftlps = (Pc - P_P) * Q_P;

== matlab function AxialPump_23a/Piston 5/Full Throttling Loss (Tank Side)/MATLAB Function ==
  data: P_T input; Pc input; P_ftlts output; Q_T input
function P_ftlts = fcn(P_T, Pc, Q_T)

P_ftlts = (P_T - Pc) * Q_T;

== matlab function AxialPump_23a/Piston 1/Pressure Side Flow Rate ==
  data: A_P input; Pc input; P_P input; Cd input; rho input; Q_P output
function Q_P = fcn(A_P, Pc, P_P, Cd, rho)

Q_P = Cd*A_P*sqrt((2/rho)*abs(Pc-P_P))*sign(Pc-P_P);

== matlab function AxialPump_23a/Piston 5/Hydrostatic Bearing Loss/MATLAB Function ==
  data: rho input; r2_r1 input; Qhbl output; r1 input; do input; d_cyl input; Cd input; Pc input
function Qhbl = fcn(rho, r2_r1, r1, do, d_cyl, Cd, Pc)

F_H = 0.25*Pc*pi*d_cyl^2;
Pp = (2*log(r2_r1)*F_H)/(((r2_r1)^2-1)*pi*r1^2);
Qhbl = 0.25*Cd*do^2*sqrt((2/rho)*abs(Pc-Pp))*sign(Pc-Pp);

== matlab function AxialPump_23a/Piston 5/Pressure Side Flow Rate ==
  data: A_P input; Pc input; P_P input; Cd input; rho input; Q_P output
function Q_P = fcn(A_P, Pc, P_P, Cd, rho)

Q_P = Cd*A_P*sqrt((2/rho)*abs(Pc-P_P))*sign(Pc-P_P);

== matlab function AxialPump_23a/Piston 5/Qleak/MATLAB Function ==
  data: Pc input; Qleak output; P_T input; d_cyl input; c input; meu input; S input
function Qleak = fcn(Pc, P_T, d_cyl, c, meu, S)

Qleak = ((0.25*pi*d_cyl^2)*c^3*(Pc-P_T))/(12*meu*S);

== matlab function AxialPump_23a/Piston 5/Tank Side Flow Rate ==
  data: A_T input; Q_T output; Pc input; P_T input; Cd input; rho input
function Q_T = fcn(A_T, Pc, P_T, Cd, rho)

Q_T = Cd*A_T*sqrt((2/rho)*abs(P_T-Pc))*sign(P_T-Pc);

== matlab function AxialPump_23a/Piston 6/Compressibility Function ==
  data: Vc_dot input; Pc_dot output; Q_T input; Q_P input; beta input; Vc input
function Pc_dot = fcn(Vc_dot, Q_T, Q_P, beta, Vc)

Pc_dot = (beta/Vc) * (Q_T - Q_P - Vc_dot);

== matlab function AxialPump_23a/Piston 6/Frictional Energy Loss/MATLAB Function ==
  data: xdot input; Pfric output; x output; Vc input; Vo input; A_cyl input; S input; c input; meu input; d_cyl input
function [Pfric, x] = fcn(xdot, Vc, Vo, A_cyl, S, c, meu, d_cyl)

x = (Vc - Vo)/A_cyl;
Pfric = (pi*d_cyl*(S-x)*meu*xdot^2)/c;

== matlab function AxialPump_23a/Piston 6/Full Throttling Loss (Pressure Side)/MATLAB Function ==
  data: Pc input; P_ftlps output; P_P input; Q_P input
function P_ftlps = fcn(Pc, P_P, Q_P)

P_ftlps = (Pc - P_P) * Q_P;

== matlab function AxialPump_23a/Piston 6/Full Throttling Loss (Tank Side)/MATLAB Function ==
  data: P_T input; Pc input; P_ftlts output; Q_T input
function P_ftlts = fcn(P_T, Pc, Q_T)

P_ftlts = (P_T - Pc) * Q_T;

== matlab function AxialPump_23a/Piston 6/Hydrostatic Bearing Loss/MATLAB Function ==
  data: rho input; r2_r1 input; Qhbl output; r1 input; do input; d_cyl input; Cd input; Pc input
function Qhbl = fcn(rho, r2_r1, r1, do, d_cyl, Cd, Pc)

F_H = 0.25*Pc*pi*d_cyl^2;
Pp = (2*log(r2_r1)*F_H)/(((r2_r1)^2-1)*pi*r1^2);
Qhbl = 0.25*Cd*do^2*sqrt((2/rho)*abs(Pc-Pp))*sign(Pc-Pp);

== matlab function AxialPump_23a/Piston 1/Eleak/MATLAB Function ==
  data: Pc input; Qleak output; P_T input; d_cyl input; c input; meu input; S input
function Qleak = fcn(Pc, P_T, d_cyl, c, meu, S)

Qleak = ((0.25*pi*d_cyl^2)*c^3*(Pc-P_T))/(12*meu*S);

== matlab function AxialPump_23a/Piston 6/Pressure Side Flow Rate ==
  data: A_P input; Pc input; P_P input; Cd input; rho input; Q_P output
function Q_P = fcn(A_P, Pc, P_P, Cd, rho)

Q_P = Cd*A_P*sqrt((2/rho)*abs(Pc-P_P))*sign(Pc-P_P);

== matlab function AxialPump_23a/Piston 6/Qleak/MATLAB Function ==
  data: Pc input; Qleak output; P_T input; d_cyl input; c input; meu input; S input
function Qleak = fcn(Pc, P_T, d_cyl, c, meu, S)

Qleak = ((0.25*pi*d_cyl^2)*c^3*(Pc-P_T))/(12*meu*S);

== matlab function AxialPump_23a/Piston 6/Tank Side Flow Rate ==
  data: A_T input; Q_T output; Pc input; P_T input; Cd input; rho input
function Q_T = fcn(A_T, Pc, P_T, Cd, rho)

Q_T = Cd*A_T*sqrt((2/rho)*abs(P_T-Pc))*sign(P_T-Pc);

== matlab function AxialPump_23a/Piston 7/Compressibility Function ==
  data: Vc_dot input; Pc_dot output; Q_T input; Q_P input; beta input; Vc input
function Pc_dot = fcn(Vc_dot, Q_T, Q_P, beta, Vc)

Pc_dot = (beta/Vc) * (Q_T - Q_P - Vc_dot);

== matlab function AxialPump_23a/Piston 7/Frictional Energy Loss/MATLAB Function ==
  data: xdot input; Pfric output; x output; Vc input; Vo input; A_cyl input; S input; c input; meu input; d_cyl input
function [Pfric, x] = fcn(xdot, Vc, Vo, A_cyl, S, c, meu, d_cyl)

x = (Vc - Vo)/A_cyl;
Pfric = (pi*d_cyl*(S-x)*meu*xdot^2)/c;

== matlab function AxialPump_23a/Piston 7/Full Throttling Loss (Pressure Side)/MATLAB Function ==
  data: Pc input; P_ftlps output; P_P input; Q_P input
function P_ftlps = fcn(Pc, P_P, Q_P)

P_ftlps = (Pc - P_P) * Q_P;

== matlab function AxialPump_23a/Piston 7/Full Throttling Loss (Tank Side)/MATLAB Function ==
  data: P_T input; Pc input; P_ftlts output; Q_T input
function P_ftlts = fcn(P_T, Pc, Q_T)

P_ftlts = (P_T - Pc) * Q_T;

== matlab function AxialPump_23a/Piston 7/Hydrostatic Bearing Loss/MATLAB Function ==
  data: rho input; r2_r1 input; Qhbl output; r1 input; do input; d_cyl input; Cd input; Pc input
function Qhbl = fcn(rho, r2_r1, r1, do, d_cyl, Cd, Pc)

F_H = 0.25*Pc*pi*d_cyl^2;
Pp = (2*log(r2_r1)*F_H)/(((r2_r1)^2-1)*pi*r1^2);
Qhbl = 0.25*Cd*do^2*sqrt((2/rho)*abs(Pc-Pp))*sign(Pc-Pp);

== matlab function AxialPump_23a/Piston 7/Pressure Side Flow Rate ==
  data: A_P input; Pc input; P_P input; Cd input; rho input; Q_P output
function Q_P = fcn(A_P, Pc, P_P, Cd, rho)

Q_P = Cd*A_P*sqrt((2/rho)*abs(Pc-P_P))*sign(Pc-P_P);

== matlab function AxialPump_23a/Piston 7/Qleak/MATLAB Function ==
  data: Pc input; Qleak output; P_T input; d_cyl input; c input; meu input; S input
function Qleak = fcn(Pc, P_T, d_cyl, c, meu, S)

Qleak = ((0.25*pi*d_cyl^2)*c^3*(Pc-P_T))/(12*meu*S);

== matlab function AxialPump_23a/Piston 7/Tank Side Flow Rate ==
  data: A_T input; Q_T output; Pc input; P_T input; Cd input; rho input
function Q_T = fcn(A_T, Pc, P_T, Cd, rho)

Q_T = Cd*A_T*sqrt((2/rho)*abs(P_T-Pc))*sign(P_T-Pc);

== matlab function AxialPump_23a/Piston 1/Frictional Energy Loss/MATLAB Function ==
  data: xdot input; Pfric output; x output; Vc input; Vo input; A_cyl input; S input; c input; meu input; d_cyl input
function [Pfric, x] = fcn(xdot, Vc, Vo, A_cyl, S, c, meu, d_cyl)

x = (Vc - Vo)/A_cyl;
Pfric = (pi*d_cyl*(S-x)*meu*xdot^2)/c;

== matlab function AxialPump_23a/Piston 8/Compressibility Function ==
  data: Vc_dot input; Pc_dot output; Q_T input; Q_P input; beta input; Vc input
function Pc_dot = fcn(Vc_dot, Q_T, Q_P, beta, Vc)

Pc_dot = (beta/Vc) * (Q_T - Q_P - Vc_dot);

== matlab function AxialPump_23a/Piston 8/Frictional Energy Loss/MATLAB Function ==
  data: xdot input; Pfric output; x output; Vc input; Vo input; A_cyl input; S input; c input; meu input; d_cyl input
function [Pfric, x] = fcn(xdot, Vc, Vo, A_cyl, S, c, meu, d_cyl)

x = (Vc - Vo)/A_cyl;
Pfric = (pi*d_cyl*(S-x)*meu*xdot^2)/c;

== matlab function AxialPump_23a/Piston 8/Full Throttling Loss (Pressure Side)/MATLAB Function ==
  data: Pc input; P_ftlps output; P_P input; Q_P input
function P_ftlps = fcn(Pc, P_P, Q_P)

P_ftlps = (Pc - P_P) * Q_P;

== matlab function AxialPump_23a/Piston 8/Full Throttling Loss (Tank Side)/MATLAB Function ==
  data: P_T input; Pc input; P_ftlts output; Q_T input
function P_ftlts = fcn(P_T, Pc, Q_T)

P_ftlts = (P_T - Pc) * Q_T;

== matlab function AxialPump_23a/Piston 8/Hydrostatic Bearing Loss/MATLAB Function ==
  data: rho input; r2_r1 input; Qhbl output; r1 input; do input; d_cyl input; Cd input; Pc input
function Qhbl = fcn(rho, r2_r1, r1, do, d_cyl, Cd, Pc)

F_H = 0.25*Pc*pi*d_cyl^2;
Pp = (2*log(r2_r1)*F_H)/(((r2_r1)^2-1)*pi*r1^2);
Qhbl = 0.25*Cd*do^2*sqrt((2/rho)*abs(Pc-Pp))*sign(Pc-Pp);

== matlab function AxialPump_23a/Piston 8/Pressure Side Flow Rate ==
  data: A_P input; Pc input; P_P input; Cd input; rho input; Q_P output
function Q_P = fcn(A_P, Pc, P_P, Cd, rho)

Q_P = Cd*A_P*sqrt((2/rho)*abs(Pc-P_P))*sign(Pc-P_P);

== matlab function AxialPump_23a/Piston 8/Qleak/MATLAB Function ==
  data: Pc input; Qleak output; P_T input; d_cyl input; c input; meu input; S input
function Qleak = fcn(Pc, P_T, d_cyl, c, meu, S)

Qleak = ((0.25*pi*d_cyl^2)*c^3*(Pc-P_T))/(12*meu*S);

== matlab function AxialPump_23a/Piston 8/Tank Side Flow Rate ==
  data: A_T input; Q_T output; Pc input; P_T input; Cd input; rho input
function Q_T = fcn(A_T, Pc, P_T, Cd, rho)

Q_T = Cd*A_T*sqrt((2/rho)*abs(P_T-Pc))*sign(P_T-Pc);

== matlab function AxialPump_23a/Piston 9/Compressibility Function ==
  data: Vc_dot input; Pc_dot output; Q_T input; Q_P input; beta input; Vc input
function Pc_dot = fcn(Vc_dot, Q_T, Q_P, beta, Vc)

Pc_dot = (beta/Vc) * (Q_T - Q_P - Vc_dot);

== matlab function AxialPump_23a/Piston 9/Frictional Energy Loss/MATLAB Function ==
  data: xdot input; Pfric output; x output; Vc input; Vo input; A_cyl input; S input; c input; meu input; d_cyl input
function [Pfric, x] = fcn(xdot, Vc, Vo, A_cyl, S, c, meu, d_cyl)

x = (Vc - Vo)/A_cyl;
Pfric = (pi*d_cyl*(S-x)*meu*xdot^2)/c;

== matlab function AxialPump_23a/Piston 9/Full Throttling Loss (Pressure Side)/MATLAB Function ==
  data: Pc input; P_ftlps output; P_P input; Q_P input
function P_ftlps = fcn(Pc, P_P, Q_P)

P_ftlps = (Pc - P_P) * Q_P;

== matlab function AxialPump_23a/Piston 9/Full Throttling Loss (Tank Side)/MATLAB Function ==
  data: P_T input; Pc input; P_ftlts output; Q_T input
function P_ftlts = fcn(P_T, Pc, Q_T)

P_ftlts = (P_T - Pc) * Q_T;

== matlab function AxialPump_23a/Piston 9/Hydrostatic Bearing Loss/MATLAB Function ==
  data: rho input; r2_r1 input; Qhbl output; r1 input; do input; d_cyl input; Cd input; Pc input
function Qhbl = fcn(rho, r2_r1, r1, do, d_cyl, Cd, Pc)

F_H = 0.25*Pc*pi*d_cyl^2;
Pp = (2*log(r2_r1)*F_H)/(((r2_r1)^2-1)*pi*r1^2);
Qhbl = 0.25*Cd*do^2*sqrt((2/rho)*abs(Pc-Pp))*sign(Pc-Pp);

== matlab function AxialPump_23a/Piston 1/Hydrostatic Bearing Loss/MATLAB Function ==
  data: rho input; r2_r1 input; Qhbl output; r1 input; do input; d_cyl input; Cd input; Pc input
function Qhbl = fcn(rho, r2_r1, r1, do, d_cyl, Cd, Pc)

F_H = 0.25*Pc*pi*d_cyl^2;
Pp = (2*log(r2_r1)*F_H)/(((r2_r1)^2-1)*pi*r1^2);
Qhbl = 0.25*Cd*do^2*sqrt((2/rho)*abs(Pc-Pp))*sign(Pc-Pp);

== matlab function AxialPump_23a/Piston 9/Pressure Side Flow Rate ==
  data: A_P input; Pc input; P_P input; Cd input; rho input; Q_P output
function Q_P = fcn(A_P, Pc, P_P, Cd, rho)

Q_P = Cd*A_P*sqrt((2/rho)*abs(Pc-P_P))*sign(Pc-P_P);

== matlab function AxialPump_23a/Piston 9/Qleak/MATLAB Function ==
  data: Pc input; Qleak output; P_T input; d_cyl input; c input; meu input; S input
function Qleak = fcn(Pc, P_T, d_cyl, c, meu, S)

Qleak = ((0.25*pi*d_cyl^2)*c^3*(Pc-P_T))/(12*meu*S);

== matlab function AxialPump_23a/Piston 9/Tank Side Flow Rate ==
  data: A_T input; Q_T output; Pc input; P_T input; Cd input; rho input
function Q_T = fcn(A_T, Pc, P_T, Cd, rho)

Q_T = Cd*A_T*sqrt((2/rho)*abs(P_T-Pc))*sign(P_T-Pc);

== matlab function AxialPump_23a/Piston 1/Full Throttling Loss (Pressure Side)/MATLAB Function ==
  data: Pc input; P_ftlps output; P_P input; Q_P input
function P_ftlps = fcn(Pc, P_P, Q_P)

P_ftlps = (Pc - P_P) * Q_P;
